simulink model "Rocket_Full_Simulation"  (R2022b)
settings: Solver=VariableStepAuto  StartTime=0.0  StopTime=5  FixedStep=0.001  EnableMultiTasking=on
model workspace (MAT data in the model file):
  Length_NC = Simulink.Parameter
  Length_NC.DataType = 'auto'
  Length_NC.Complexity = 'real'
  Length_NC.Dimensions = [0 0]
undefined symbols (not defined in the file): sigbuilder_block
libraries: simulink_extras x3, simulink x3, sharedtransform x2, mspsensorlib x1, aerolibatmos2 x1, vrlib x1
settings Model: Creator=Poseidon  LastModifiedBy=Poseidon
settings SolverCC: MaxConsecutiveMinStep=3  ZeroCrossAlgorithm=Adaptive  AutoInsertRateTranBlk=on
settings DataIOCC: Refine=2
settings DebuggingCC: ReadBeforeWriteMsg=DisableAll  WriteAfterWriteMsg=DisableAll  WriteAfterReadMsg=DisableAll  MaskedZcDiagnostic=none  IgnoredZcDiagnostic=none  MultiTaskDSMMsg=none
settings ModelReferenceCC: UpdateModelReferenceTargets=IfOutOfDate  EnableRefExpFcnMdlSchedulingChecks=on
settings SFSimCC: SFSimEcho=off

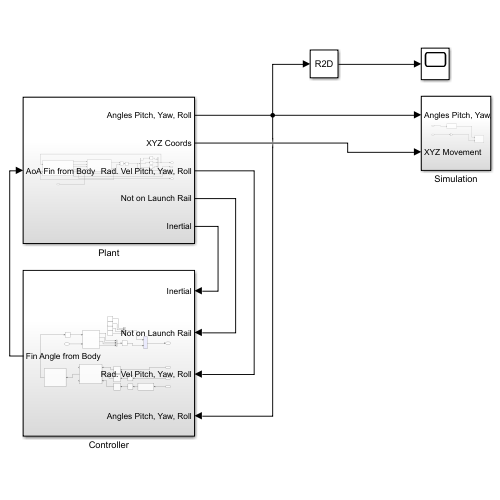
[thumbnail: Simulink's stored preview of the top-level diagram]
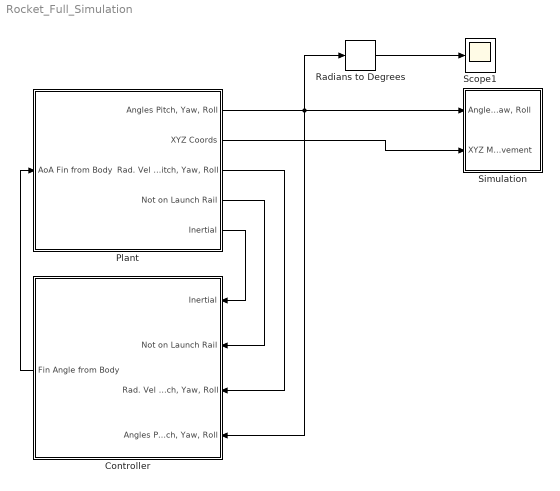
== system Rocket_Full_Simulation ==
  Controller : Subsystem
  Plant : Subsystem
  Radians to Degrees : simulink_extras/Transformations/Radians to Degrees
  Scope1 : Scope
  Simulation : Subsystem
  wires:
  Plant/2(XYZ Coords) -> Simulation/2(XYZ Movement)
  Plant/4(Not on Launch Rail) -> Controller/2(Not on Launch Rail)
  Plant/5(Inertial) -> Controller/1(Inertial)
  Controller/1(Fin Angle from Body) -> Plant/1(AoA Fin from Body)
  Plant/1("Angles Pitch, Yaw, Roll") -> Controller/4("Angles Pitch, Yaw, Roll"), Simulation/1("Angles Pitch, Yaw, Roll"), Radians to Degrees/1
  Plant/3("Rad. Vel Pitch, Yaw, Roll") -> Controller/3("Rad. Vel Pitch, Yaw, Roll")
  Radians to Degrees/1 -> Scope1/1

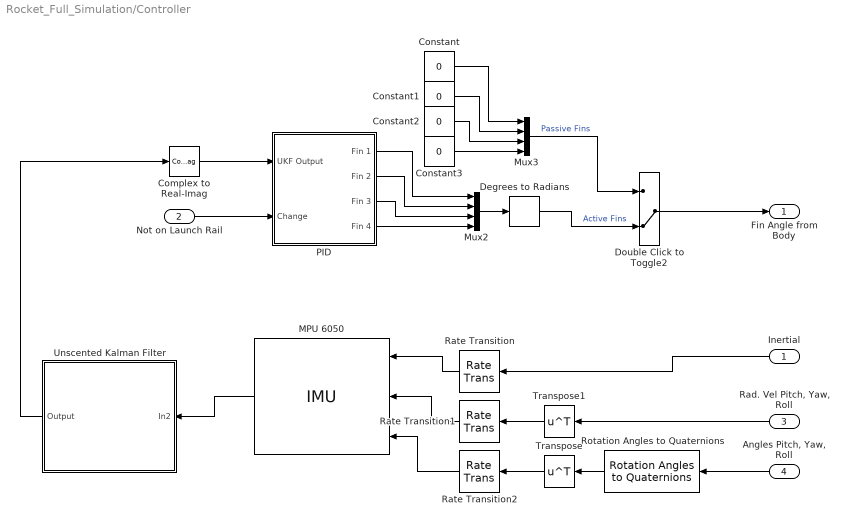
== system Rocket_Full_Simulation/Controller ==
  Inertial : Inport
  Not on Launch Rail : Inport  Port=2
  "Rad. Vel Pitch, Yaw, Roll" : Inport  Port=3
  "Angles Pitch, Yaw, Roll" : Inport  Port=4
  Complex to Real-Imag : ComplexToRealImag  Output=Real
  Constant{,1..3} (4 alike) : Constant  Value=0
  Degrees to Radians : simulink_extras/Transformations/Degrees to Radians
  Double Click to Toggle2 : ManualSwitch  CurrentSetting=0
  MPU 6050 : mspsensorlib/IMU  DispRefFrame=NED  Temperature=25  MagneticFieldNED=[ 27.5550, -2.4169, -16.0849 ]  MagneticFieldENU=[ -2.4169, 27.5550, 16.0849 ]  SeedDouble=67  SimulateUsing=Code generation  AccelParamsMeasurementRange=160  AccelParamsResolution=0.00479  AccelParamsConstantBias=[ 0, 0, 0 ]  AccelParamsAxesMisalignment=[ 100, 0, 0; 0, 100, 0; 0, 0, 100 ]  AccelParamsNoiseDensity=[ 0, 0, 0 ]  AccelParamsBiasInstability=[ 0, 0, 0 ]  AccelParamsRandomWalk=[ 0, 0, 0 ]  AccelParamsTemperatureBias=[ 0, 0, 0 ]  AccelParamsTemperatureScaleFactor=[ 0, 0, 0 ]  GyroParamsMeasurementRange=4.36332  GyroParamsResolution=0.000133157958984  GyroParamsConstantBias=[ 0, 0, 0 ]  GyroParamsAxesMisalignment=[ 100, 0, 0; 0, 100, 0; 0, 0, 100 ]  GyroParamsAccelerationBias=[ 0, 0, 0 ]  GyroParamsNoiseDensity=[ 5.24*10^-5, 5.24*10^-5, 5.24*10^-5 ]  GyroParamsBiasInstability=[ 2.09*10^-5, 2.09*10^-5, 2.09*10^-5 ]  GyroParamsRandomWalk=[ 0, 0, 0 ]  GyroParamsTemperatureBias=[ 0, 0, 0 ]  GyroParamsTemperatureScaleFactor=[ 0, 0, 0 ]  MagParamsMeasurementRange=Inf  MagParamsResolution=0  MagParamsConstantBias=[ 0, 0, 0 ]  MagParamsAxesMisalignment=[ 100, 0, 0; 0, 100, 0; 0, 0, 100 ]  MagParamsNoiseDensity=[ 0, 0, 0 ]  MagParamsBiasInstability=[ 0, 0, 0 ]  MagParamsRandomWalk=[ 0, 0, 0 ]  MagParamsTemperatureBias=[ 0, 0, 0 ]  MagParamsTemperatureScaleFactor=[ 0, 0, 0 ]
  Mux2 : Mux
  Mux3 : Mux
  PID : Subsystem
  Rate Transition : RateTransition  OutPortSampleTime=0.001
  Rate Transition1 : RateTransition  OutPortSampleTime=0.001
  Rate Transition2 : RateTransition  OutPortSampleTime=0.001
  Rotation Angles to Quaternions : sharedtransform/Rotation Angles to Quaternions  rotationOrder=YZX  aMode=aMode
  Transpose : Math  Operator=transpose
  Transpose1 : Math  Operator=transpose
  Unscented Kalman Filter : Subsystem
  Fin Angle from Body : Outport
  wires:
  Constant3/1 -> Mux3/4
  PID/1(Fin 1) -> Mux2/1
  Mux2/1 -> Degrees to Radians/1
  PID/4(Fin 4) -> Mux2/4
  Constant2/1 -> Mux3/3
  Constant/1 -> Mux3/1
  PID/3(Fin 3) -> Mux2/3
  PID/2(Fin 2) -> Mux2/2
  Mux3/1 -> Double Click to Toggle2/1  "Passive Fins"
  Constant1/1 -> Mux3/2
  Complex to Real-Imag/1 -> PID/1(UKF Output)
  Unscented Kalman Filter/1(Output) -> Complex to Real-Imag/1
  Degrees to Radians/1 -> Double Click to Toggle2/2  "Active Fins"
  Double Click to Toggle2/1 -> Fin Angle from Body/1
  Not on Launch Rail/1 -> PID/2(Change)
  "Rad. Vel Pitch, Yaw, Roll"/1 -> Transpose1/1
  "Angles Pitch, Yaw, Roll"/1 -> Rotation Angles to Quaternions/1
  MPU 6050/2 -> Unscented Kalman Filter/1(In2)
  Inertial/1 -> Rate Transition/1
  Transpose/1 -> Rate Transition2/1
  Rate Transition2/1 -> MPU 6050/3
  Rate Transition/1 -> MPU 6050/1
  Rotation Angles to Quaternions/1 -> Transpose/1
  Rate Transition1/1 -> MPU 6050/2
  Transpose1/1 -> Rate Transition1/1

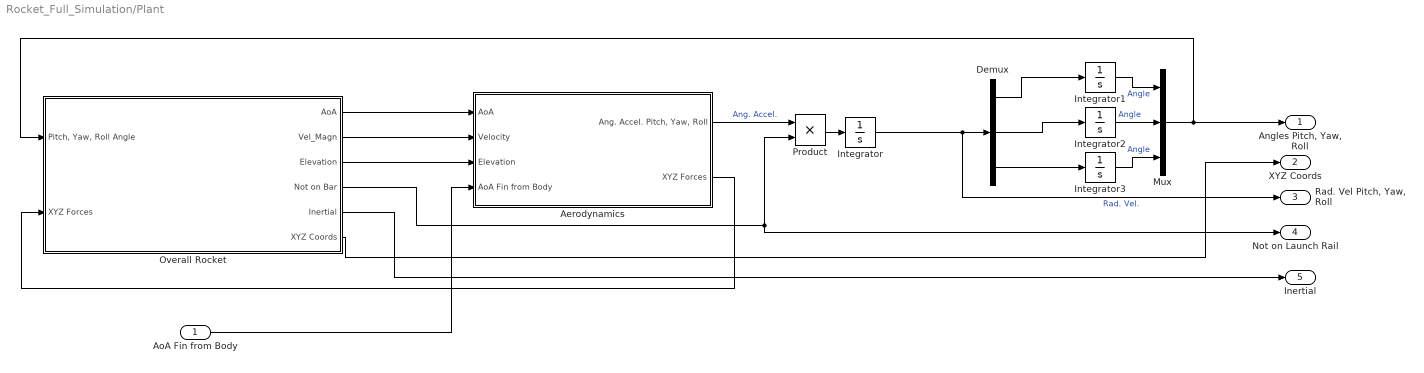
== system Rocket_Full_Simulation/Plant ==
  AoA Fin from Body : Inport
  Aerodynamics : Subsystem
  Demux : Demux  Outputs=3
  Integrator : Integrator
  Integrator1 : Integrator  InitialCondition=0*(pi/180)
  Integrator2 : Integrator
  Integrator3 : Integrator
  Mux : Mux  Inputs=3
  Overall Rocket : Subsystem
  Product : Product
  "Angles Pitch, Yaw, Roll" : Outport
  XYZ Coords : Outport  Port=2
  "Rad. Vel Pitch, Yaw, Roll" : Outport  Port=3
  Not on Launch Rail : Outport  Port=4
  Inertial : Outport  Port=5
  wires:
  Integrator2/1 -> Mux/2  "Angle"
  Product/1 -> Integrator/1
  Integrator/1 -> "Rad. Vel Pitch, Yaw, Roll"/1, Demux/1  "Rad. Vel."
  Demux/2 -> Integrator2/1
  Demux/1 -> Integrator1/1
  Integrator3/1 -> Mux/3  "Angle"
  Demux/3 -> Integrator3/1
  Integrator1/1 -> Mux/1  "Angle"
  Mux/1 -> Overall Rocket/1("Pitch, Yaw, Roll Angle"), "Angles Pitch, Yaw, Roll"/1
  AoA Fin from Body/1 -> Aerodynamics/4(AoA Fin from Body)
  Overall Rocket/1(AoA) -> Aerodynamics/1(AoA)
  Overall Rocket/5(Inertial) -> Inertial/1
  Overall Rocket/2(Vel_Magn) -> Aerodynamics/2(Velocity)
  Overall Rocket/3(Elevation) -> Aerodynamics/3(Elevation)
  Overall Rocket/4(Not on Bar) -> Not on Launch Rail/1, Product/2
  Aerodynamics/1("Ang. Accel. Pitch, Yaw, Roll") -> Product/1  "Ang. Accel."
  Aerodynamics/2(XYZ Forces) -> Overall Rocket/2(XYZ Forces)
  Overall Rocket/6(XYZ Coords) -> XYZ Coords/1

== system Rocket_Full_Simulation/Simulation ==
  note: Convert to coordinates for simulation
  "Angles Pitch, Yaw, Roll" : Inport
  XYZ Movement : Inport  Port=2
  MATLAB Function : MATLAB Function  TreatAsAtomicUnit=on
  Multiply : Gain  Gain=0
  VR Sink : vrlib/VR Sink  InstantiateOnLoad=on  SampleTime=0.1  ViewEnable=on  RemoteChange=off  RemoteView=off  FieldsWritten=node_Transform.rotation.4.1.1.double#node_Transform.translation.3.1.1.double  WorldFileName=C:\Users\Trenton VerKuilen\OneDrive - lmu.edu\School\Capstone\2Stage_Rocket.wrl  AutoView=off  VideoDimensions=[]  AllowVariableSize=off
  wires:
  XYZ Movement/1 -> Multiply/1
  Multiply/1 -> VR Sink/2
  "Angles Pitch, Yaw, Roll"/1 -> MATLAB Function/1(Angles)
  MATLAB Function/1(Rotation) -> VR Sink/1

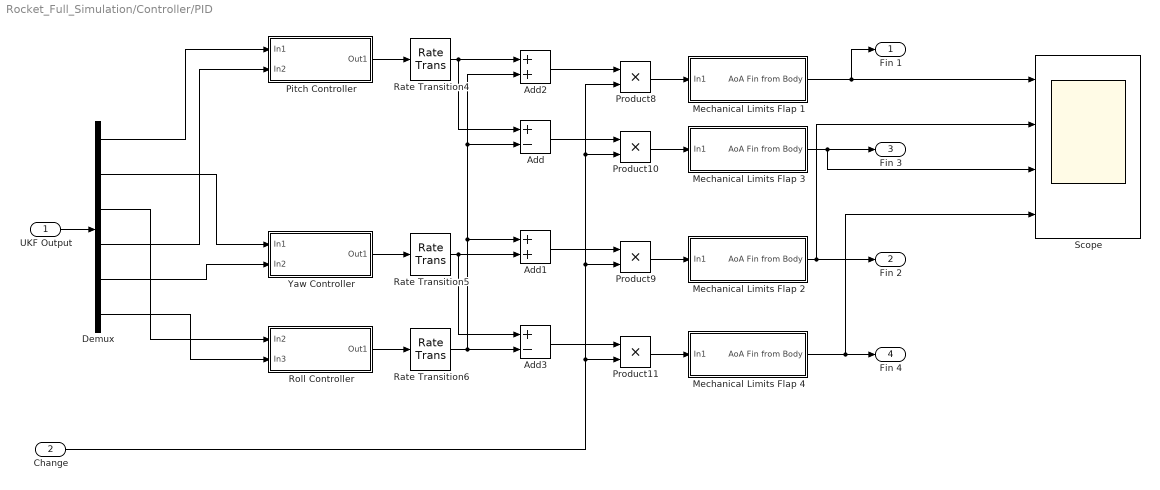
== system Rocket_Full_Simulation/Controller/PID ==
  UKF Output : Inport
  Change : Inport  Port=2
  Add : Sum  Inputs=+-
  Add1 : Sum
  Add2 : Sum
  Add3 : Sum  Inputs=+-
  Demux : Demux  Outputs=6
  Mechanical Limits Flap 1 : Subsystem
  Mechanical Limits Flap 2 : Subsystem
  Mechanical Limits Flap 3 : Subsystem
  Mechanical Limits Flap 4 : Subsystem
  Pitch Controller : Subsystem
  Product{8..11} (4 alike) : Product
  Rate Transition4 : RateTransition
  Rate Transition5 : RateTransition
  Rate Transition6 : RateTransition
  Roll Controller : Subsystem
  Scope : Scope  NumInputPorts=4
  Yaw Controller : Subsystem
  Fin 1 : Outport
  Fin 2 : Outport  Port=2
  Fin 3 : Outport  Port=3
  Fin 4 : Outport  Port=4
  wires:
  UKF Output/1 -> Demux/1
  Demux/5 -> Yaw Controller/2(In2)
  Demux/2 -> Yaw Controller/1(In1)
  Demux/1 -> Pitch Controller/1(In1)
  Pitch Controller/1(Out1) -> Rate Transition4/1
  Demux/3 -> Roll Controller/1(In2)
  Demux/4 -> Pitch Controller/2(In2)
  Demux/6 -> Roll Controller/2(In3)
  Yaw Controller/1(Out1) -> Rate Transition5/1
  Roll Controller/1(Out1) -> Rate Transition6/1
  Rate Transition4/1 -> Add/1, Add2/1
  Rate Transition5/1 -> Add3/1, Add1/2
  Rate Transition6/1 -> Add2/2, Add/2, Add1/1, Add3/2
  Add2/1 -> Product8/1
  Add/1 -> Product10/1
  Add1/1 -> Product9/1
  Mechanical Limits Flap 2/1(AoA Fin from Body) -> Scope/2, Fin 2/1
  Change/1 -> Product8/2, Product10/2, Product9/2, Product11/2
  Add3/1 -> Product11/1
  Product8/1 -> Mechanical Limits Flap 1/1(In1)
  Product9/1 -> Mechanical Limits Flap 2/1(In1)
  Product10/1 -> Mechanical Limits Flap 3/1(In1)
  Product11/1 -> Mechanical Limits Flap 4/1(In1)
  Mechanical Limits Flap 1/1(AoA Fin from Body) -> Fin 1/1, Scope/1
  Mechanical Limits Flap 3/1(AoA Fin from Body) -> Scope/3, Fin 3/1
  Mechanical Limits Flap 4/1(AoA Fin from Body) -> Scope/4, Fin 4/1

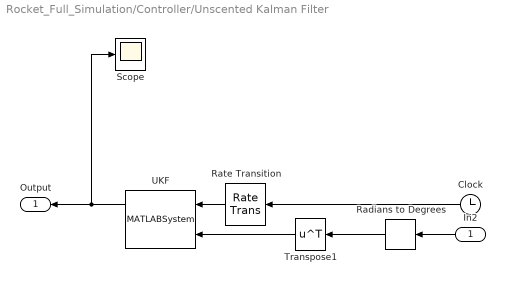
== system Rocket_Full_Simulation/Controller/Unscented Kalman Filter ==
  In2 : Inport
  Clock : Clock
  Radians to Degrees : simulink_extras/Transformations/Radians to Degrees
  Rate Transition : RateTransition  OutPortSampleTime=0.001
  Scope : Scope
  Transpose1 : Math  Operator=transpose
  UKF : MATLABSystem  System=UKF  kappa=0.0  alfa=0.001  beta=2.0  x_0=0  Q_=0.1  R_=0.1  SimulateUsing=Code generation
      mask Type: UKF
      mask Display:
      | disp('UKF');
      | port_label('input',1,'time');
      | port_label('input',2,'z');
      | port_label('output',1,'y');
      | port_label('output',2,'P');
  Output : Outport
  wires:
  UKF/1 -> Scope/1, Output/1
  In2/1 -> Radians to Degrees/1
  Radians to Degrees/1 -> Transpose1/1
  Transpose1/1 -> UKF/2
  Clock/1 -> Rate Transition/1
  Rate Transition/1 -> UKF/1

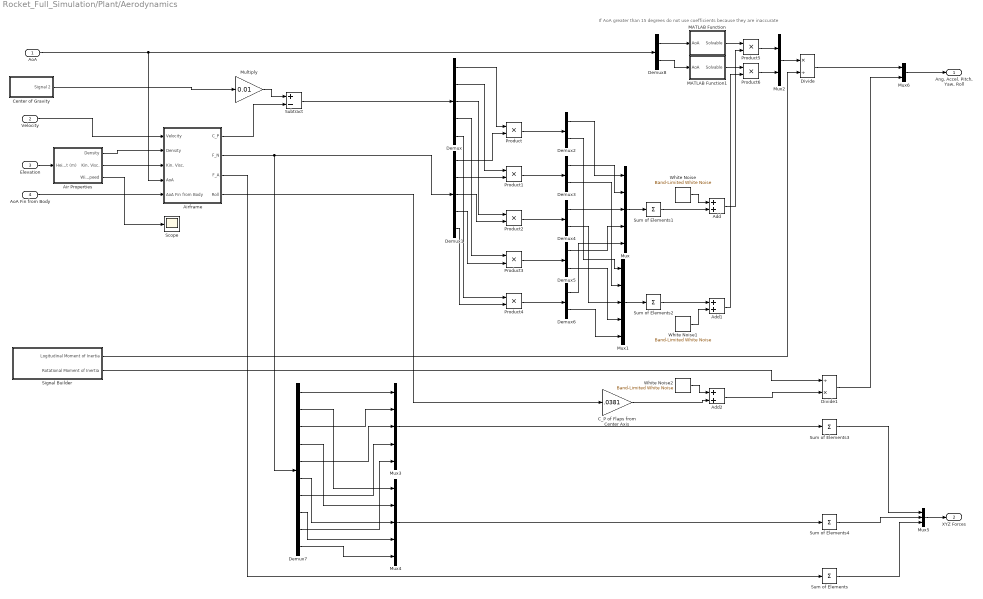
== system Rocket_Full_Simulation/Plant/Aerodynamics ==
  note: If AoA greater than 15 degrees do not use coefficients because they are inaccurate
  AoA : Inport
  Velocity : Inport  Port=2
  Elevation : Inport  Port=3
  AoA Fin from Body : Inport  Port=4
  Add : Sum
  Add1 : Sum
  Add2 : Sum
  Air Properties : Subsystem
  Airframe : Subsystem
  C_P of Flaps from Center Axis : Gain  Gain=.0381
  Center of Gravity : Subsystem  Tag=STV Subsys  LoadFcn=sigbuilder_block('load');  StartFcn=sigbuilder_block('start');  StopFcn=sigbuilder_block('stop');  ClipboardFcn=sigbuilder_block('clipboard');  mask(Sigbuilder block){tuvar=[0:10]}
      mask help: Simulink:masks:SigbuilderBlock_MD
      mask init:
      | if ~strcmp(get_param(bdroot(gcbh),'SimulationStatus'),'stopped') tuvar = sigbuilder_block('maskInit'); end
      settings: CopyFcn=sigbuilder_block('copy');  DeleteFcn=sigbuilder_block('delete');  ModelCloseFcn=sigbuilder_block('modelClose');  PreSaveFcn=sigbuilder_block('preSave');  PauseFcn=sigbuilder_block('pause');  ContinueFcn=sigbuilder_block('continue');  NameChangeFcn=sigbuilder_block('namechange');  OpenFcn=sigbuilder_block('open',[309.6 144.6 550.8 400.2 ]);  CloseFcn=sigbuilder_block('close');
      mask Display: plot(0, 0, 100, 100,[2, 2, 32, 32, 2], [68, 8, 8, 68, 68],[32, 2], [38, 38], [32, 19, 2],[53, 60, 44], [32, 17, 17, 2],[16, 16, 31, 31]);txt = getActiveGroup(gcbh);text(2, 100, txt,'verticalAlignment', 'top');
  Demux : Demux  Outputs=5
  Demux1 : Demux  Outputs=5
  Demux{2..6,8} (6 alike) : Demux  Outputs=2
  Demux7 : Demux  Outputs=10
  Divide : Product  Inputs=*/
  Divide1 : Product  Inputs=/*
  MATLAB Function : MATLAB Function  TreatAsAtomicUnit=on
  MATLAB Function1 : MATLAB Function  TreatAsAtomicUnit=on
  Multiply : Gain  Gain=0.01
  Mux{,1,3..4} (4 alike) : Mux  Inputs=5
  Mux2 : Mux  Inputs=2
  Mux5 : Mux  Inputs=3
  Mux6 : Mux  Inputs=2
  Product{,1..6} (7 alike) : Product
  Scope : Scope
  Signal Builder : Subsystem  Tag=STV Subsys  LoadFcn=sigbuilder_block('load');  StartFcn=sigbuilder_block('start');  StopFcn=sigbuilder_block('stop');  ClipboardFcn=sigbuilder_block('clipboard');  mask(Sigbuilder block){tuvar=[0:10]}
      mask help: Simulink:masks:SigbuilderBlock_MD
      mask init:
      | if ~strcmp(get_param(bdroot(gcbh),'SimulationStatus'),'stopped') tuvar = sigbuilder_block('maskInit'); end
      settings: CopyFcn=sigbuilder_block('copy');  DeleteFcn=sigbuilder_block('delete');  ModelCloseFcn=sigbuilder_block('modelClose');  PreSaveFcn=sigbuilder_block('preSave');  PauseFcn=sigbuilder_block('pause');  ContinueFcn=sigbuilder_block('continue');  NameChangeFcn=sigbuilder_block('namechange');  OpenFcn=sigbuilder_block('open',[375 140.4 550.8 400.2 ]);  CloseFcn=sigbuilder_block('close');
      mask Display: plot(0, 0, 100, 100,[2, 2, 32, 32, 2], [68, 8, 8, 68, 68],[32, 2], [38, 38], [32, 19, 2],[53, 60, 44], [32, 17, 17, 2],[16, 16, 31, 31]);txt = getActiveGroup(gcbh);text(2, 100, txt,'verticalAlignment', 'top');
  Subtract : Sum  Inputs=+-
  Sum of Elements{,1..4} (5 alike) : Sum  Inputs=+
  White Noise : simulink/Sources/Band-Limited White Noise  Cov=[0.005]  Ts=0.5  seed=[12345]
  White Noise1 : simulink/Sources/Band-Limited White Noise  Cov=[0.005]  Ts=0.5  seed=[84932]
  White Noise2 : simulink/Sources/Band-Limited White Noise  Cov=[0.000001]  Ts=0.5  seed=[86986]
  "Ang. Accel. Pitch, Yaw, Roll" : Outport
  XYZ Forces : Outport  Port=2
  wires:
  Airframe/1(C_P) -> Subtract/2
  Elevation/1 -> Air Properties/1(Height (m))
  Demux7/5 -> Mux3/3
  Center of Gravity/1(Signal 2) -> Multiply/1
  C_P of Flaps from Center Axis/1 -> Add2/2
  AoA Fin from Body/1 -> Airframe/5(AoA Fin from Body)
  AoA/1 -> Demux8/1, Airframe/4(AoA)
  Air Properties/3(Wind Speed) -> Scope/1
  Demux/3 -> Product2/1
  Demux7/8 -> Mux4/4
  Demux8/1 -> MATLAB Function/1(AoA)
  Velocity/1 -> Airframe/1(Velocity)
  Air Properties/2(Kin. Visc.) -> Airframe/3(Kin. Visc.)
  Demux3/2 -> Mux1/2
  Demux/5 -> Product4/1
  Air Properties/1(Density) -> Airframe/2(Density)
  Multiply/1 -> Subtract/1
  Sum of Elements4/1 -> Mux5/2
  Airframe/2(F_N) -> Demux1/1, Demux7/1
  Airframe/3(F_A) -> Sum of Elements/1
  Airframe/4(Roll) -> C_P of Flaps from Center Axis/1
  Demux7/2 -> Mux4/1
  Subtract/1 -> Demux/1
  Demux7/1 -> Mux3/1
  Demux7/3 -> Mux3/2
  Demux7/4 -> Mux4/2
  Demux7/6 -> Mux4/3
  Demux6/2 -> Mux1/5
  Demux7/7 -> Mux3/4
  Demux7/9 -> Mux3/5
  Product4/1 -> Demux6/1
  Mux3/1 -> Sum of Elements3/1
  Demux7/10 -> Mux4/5
  Demux1/4 -> Product3/2
  Mux1/1 -> Sum of Elements2/1
  Add2/1 -> Divide1/2
  White Noise2/1 -> Add2/1
  Demux/1 -> Product/1
  Demux/2 -> Product1/1
  Sum of Elements3/1 -> Mux5/1
  Demux/4 -> Product3/1
  Demux4/1 -> Mux/3
  Demux1/1 -> Product/2
  Demux1/2 -> Product1/2
  Demux1/3 -> Product2/2
  Product3/1 -> Demux5/1
  Demux1/5 -> Product4/2
  Mux4/1 -> Sum of Elements4/1
  Signal Builder/1(Logitudinal Moment of Inertia) -> Divide/2
  White Noise/1 -> Add/1
  Signal Builder/2(Rotational Moment of Inertia) -> Divide1/1
  Demux3/1 -> Mux/2
  Product/1 -> Demux2/1
  Product1/1 -> Demux3/1
  Demux5/1 -> Mux/4
  Product2/1 -> Demux4/1
  Divide1/1 -> Mux6/2
  Demux2/1 -> Mux/1
  Demux2/2 -> Mux1/1
  Demux4/2 -> Mux1/3
  Demux5/2 -> Mux1/4
  Demux6/1 -> Mux/5
  Mux/1 -> Sum of Elements1/1
  Demux8/2 -> MATLAB Function1/1(AoA)
  Sum of Elements1/1 -> Add/2
  Sum of Elements2/1 -> Add1/1
  White Noise1/1 -> Add1/2
  MATLAB Function/1(Solvable) -> Product5/1
  Add/1 -> Product5/2
  MATLAB Function1/1(Solvable) -> Product6/1
  Add1/1 -> Product6/2
  Product5/1 -> Mux2/1
  Product6/1 -> Mux2/2
  Mux2/1 -> Divide/1
  Mux5/1 -> XYZ Forces/1
  Mux6/1 -> "Ang. Accel. Pitch, Yaw, Roll"/1
  Divide/1 -> Mux6/1
  Sum of Elements/1 -> Mux5/3

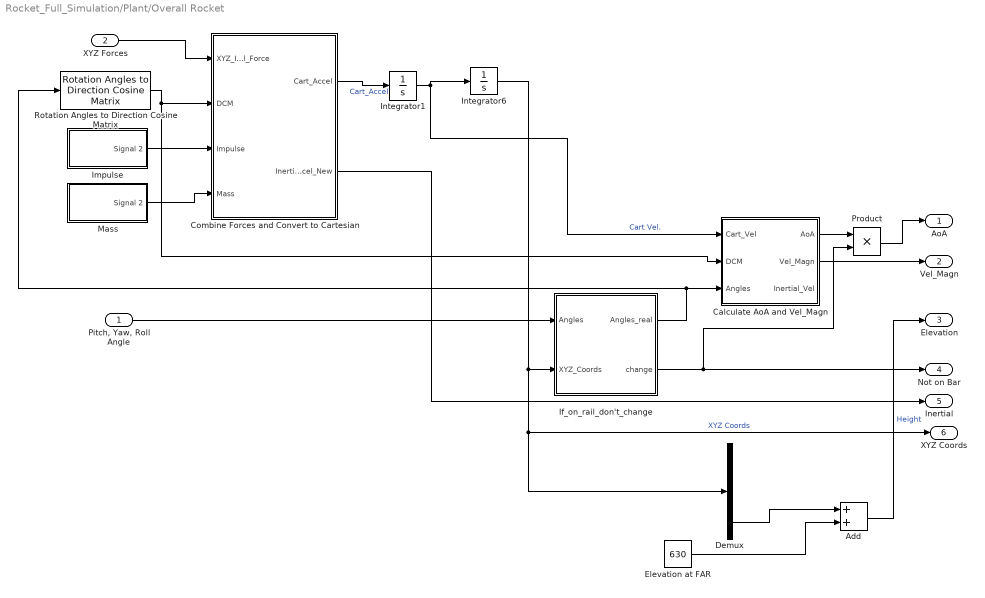
== system Rocket_Full_Simulation/Plant/Overall Rocket ==
  "Pitch, Yaw, Roll Angle" : Inport
  XYZ Forces : Inport  Port=2
  Add : Sum
  Calculate AoA and Vel_Magn : MATLAB Function  TreatAsAtomicUnit=on
  Combine Forces and Convert to Cartesian : MATLAB Function  TreatAsAtomicUnit=on
  Demux : Demux  Outputs=3
  Elevation at FAR : Constant  Value=630
  If_on_rail_don't_change : MATLAB Function  TreatAsAtomicUnit=on
  Impulse : Subsystem  Tag=STV Subsys  LoadFcn=sigbuilder_block('load');  StartFcn=sigbuilder_block('start');  StopFcn=sigbuilder_block('stop');  ClipboardFcn=sigbuilder_block('clipboard');  mask(Sigbuilder block){tuvar=[0:10]}
      mask help: Simulink:masks:SigbuilderBlock_MD
      mask init:
      | if ~strcmp(get_param(bdroot(gcbh),'SimulationStatus'),'stopped') tuvar = sigbuilder_block('maskInit'); end
      settings: CopyFcn=sigbuilder_block('copy');  DeleteFcn=sigbuilder_block('delete');  ModelCloseFcn=sigbuilder_block('modelClose');  PreSaveFcn=sigbuilder_block('preSave');  PauseFcn=sigbuilder_block('pause');  ContinueFcn=sigbuilder_block('continue');  NameChangeFcn=sigbuilder_block('namechange');  OpenFcn=sigbuilder_block('open',[396 -4.2 574.2 590.4 ]);  CloseFcn=sigbuilder_block('close');
      mask Display: plot(0, 0, 100, 100,[2, 2, 32, 32, 2], [68, 8, 8, 68, 68],[32, 2], [38, 38], [32, 19, 2],[53, 60, 44], [32, 17, 17, 2],[16, 16, 31, 31]);txt = getActiveGroup(gcbh);text(2, 100, txt,'verticalAlignment', 'top');
  Integrator1 : Integrator  IgnoreLimit=on
  Integrator6 : Integrator
  Mass : Subsystem  Tag=STV Subsys  LoadFcn=sigbuilder_block('load');  StartFcn=sigbuilder_block('start');  StopFcn=sigbuilder_block('stop');  ClipboardFcn=sigbuilder_block('clipboard');  mask(Sigbuilder block){tuvar=[0:10]}
      mask help: Simulink:masks:SigbuilderBlock_MD
      mask init:
      | if ~strcmp(get_param(bdroot(gcbh),'SimulationStatus'),'stopped') tuvar = sigbuilder_block('maskInit'); end
      settings: CopyFcn=sigbuilder_block('copy');  DeleteFcn=sigbuilder_block('delete');  ModelCloseFcn=sigbuilder_block('modelClose');  PreSaveFcn=sigbuilder_block('preSave');  PauseFcn=sigbuilder_block('pause');  ContinueFcn=sigbuilder_block('continue');  NameChangeFcn=sigbuilder_block('namechange');  OpenFcn=sigbuilder_block('open',[424.8 154.2 550.8 400.2 ]);  CloseFcn=sigbuilder_block('close');
      mask Display: plot(0, 0, 100, 100,[2, 2, 32, 32, 2], [68, 8, 8, 68, 68],[32, 2], [38, 38], [32, 19, 2],[53, 60, 44], [32, 17, 17, 2],[16, 16, 31, 31]);txt = getActiveGroup(gcbh);text(2, 100, txt,'verticalAlignment', 'top');
  Product : Product
  Rotation Angles to Direction Cosine Matrix : sharedtransform/Rotation Angles to Direction Cosine Matrix  rotationOrder=YZX  aMode=aMode
  AoA : Outport
  Vel_Magn : Outport  Port=2
  Elevation : Outport  Port=3
  Not on Bar : Outport  Port=4
  Inertial : Outport  Port=5
  XYZ Coords : Outport  Port=6
  wires:
  XYZ Forces/1 -> Combine Forces and Convert to Cartesian/1(XYZ_Inertial_Force)
  Impulse/1(Signal 2) -> Combine Forces and Convert to Cartesian/3(Impulse)
  Rotation Angles to Direction Cosine Matrix/1 -> Calculate AoA and Vel_Magn/2(DCM), Combine Forces and Convert to Cartesian/2(DCM)
  Integrator1/1 -> Integrator6/1, Calculate AoA and Vel_Magn/1(Cart_Vel)  "Cart Vel."
  Mass/1(Signal 2) -> Combine Forces and Convert to Cartesian/4(Mass)
  Combine Forces and Convert to Cartesian/2(Inertial_Accel_New) -> Inertial/1
  Combine Forces and Convert to Cartesian/1(Cart_Accel) -> Integrator1/1  "Cart_Accel"
  Integrator6/1 -> Demux/1, XYZ Coords/1, If_on_rail_don't_change/2(XYZ_Coords)  "XYZ Coords"
  "Pitch, Yaw, Roll Angle"/1 -> If_on_rail_don't_change/1(Angles)
  Demux/3 -> Add/1
  Elevation at FAR/1 -> Add/2
  If_on_rail_don't_change/1(Angles_real) -> Rotation Angles to Direction Cosine Matrix/1, Calculate AoA and Vel_Magn/3(Angles)
  If_on_rail_don't_change/2(change) -> Product/2, Not on Bar/1
  Add/1 -> Elevation/1  "Height"
  Calculate AoA and Vel_Magn/2(Vel_Magn) -> Vel_Magn/1
  Calculate AoA and Vel_Magn/1(AoA) -> Product/1
  Product/1 -> AoA/1

== system Rocket_Full_Simulation/Controller/PID/Mechanical Limits Flap 1 ==
  In1 : Inport
  Integrator Limited : Integrator  LimitOutput=on  UpperSaturationLimit=15  LowerSaturationLimit=-15
  Rate Limit : Saturate  UpperLimit=857.14  LowerLimit=-857.14
  Servo Gain : Gain  Gain=6
  Sum2 : Sum  Inputs=|+-
  AoA Fin from Body : Outport
  wires:
  Sum2/1 -> Servo Gain/1
  Servo Gain/1 -> Rate Limit/1
  Rate Limit/1 -> Integrator Limited/1
  In1/1 -> Sum2/1
  Integrator Limited/1 -> AoA Fin from Body/1, Sum2/2

== system Rocket_Full_Simulation/Controller/PID/Mechanical Limits Flap 2 ==
  In1 : Inport
  Integrator Limited : Integrator  LimitOutput=on  UpperSaturationLimit=15  LowerSaturationLimit=-15
  Rate Limit : Saturate  UpperLimit=857.14  LowerLimit=-857.14
  Servo Gain : Gain  Gain=6
  Sum2 : Sum  Inputs=|+-
  AoA Fin from Body : Outport
  wires:
  Sum2/1 -> Servo Gain/1
  Servo Gain/1 -> Rate Limit/1
  Rate Limit/1 -> Integrator Limited/1
  In1/1 -> Sum2/1
  Integrator Limited/1 -> AoA Fin from Body/1, Sum2/2

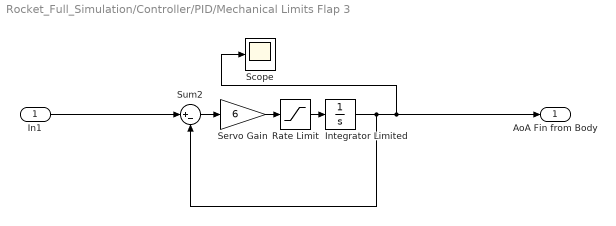
== system Rocket_Full_Simulation/Controller/PID/Mechanical Limits Flap 3 ==
  In1 : Inport
  Integrator Limited : Integrator  LimitOutput=on  UpperSaturationLimit=15  LowerSaturationLimit=-15
  Rate Limit : Saturate  UpperLimit=857.14  LowerLimit=-857.14
  Scope : Scope
  Servo Gain : Gain  Gain=6
  Sum2 : Sum  Inputs=|+-
  AoA Fin from Body : Outport
  wires:
  Sum2/1 -> Servo Gain/1
  Servo Gain/1 -> Rate Limit/1
  Rate Limit/1 -> Integrator Limited/1
  In1/1 -> Sum2/1
  Integrator Limited/1 -> Scope/1, AoA Fin from Body/1, Sum2/2

== system Rocket_Full_Simulation/Controller/PID/Mechanical Limits Flap 4 ==
  In1 : Inport
  Integrator Limited : Integrator  LimitOutput=on  UpperSaturationLimit=15  LowerSaturationLimit=-15
  Rate Limit : Saturate  UpperLimit=857.14  LowerLimit=-857.14
  Servo Gain : Gain  Gain=6
  Sum2 : Sum  Inputs=|+-
  AoA Fin from Body : Outport
  wires:
  Sum2/1 -> Servo Gain/1
  Servo Gain/1 -> Rate Limit/1
  Rate Limit/1 -> Integrator Limited/1
  In1/1 -> Sum2/1
  Integrator Limited/1 -> AoA Fin from Body/1, Sum2/2

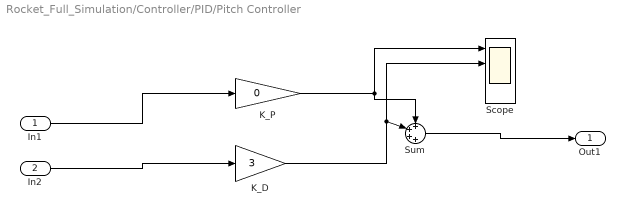
== system Rocket_Full_Simulation/Controller/PID/Pitch Controller ==
  In1 : Inport
  In2 : Inport  Port=2
  K_D : Gain  Gain=3
  K_P : Gain  Gain=0
  Scope : Scope  NumInputPorts=4
  Sum : Sum  Inputs=++++
  Out1 : Outport
  wires:
  In2/1 -> K_D/1
  In1/1 -> K_P/1
  K_P/1 -> Sum/1, Scope/1
  K_D/1 -> Scope/2, Sum/2
  Sum/1 -> Out1/1

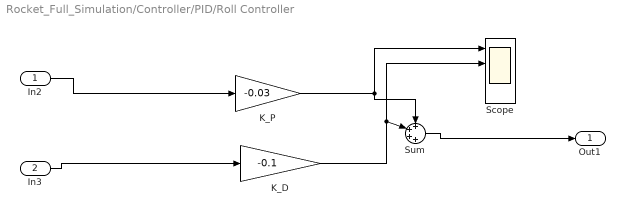
== system Rocket_Full_Simulation/Controller/PID/Roll Controller ==
  In2 : Inport
  In3 : Inport  Port=2
  K_D : Gain  Gain=-0.1
  K_P : Gain  Gain=-0.03
  Scope : Scope  NumInputPorts=4
  Sum : Sum  Inputs=++++
  Out1 : Outport
  wires:
  In3/1 -> K_D/1
  K_P/1 -> Sum/1, Scope/1
  K_D/1 -> Scope/2, Sum/2
  In2/1 -> K_P/1
  Sum/1 -> Out1/1

== system Rocket_Full_Simulation/Controller/PID/Yaw Controller ==
  In1 : Inport
  In2 : Inport  Port=2
  K_D : Gain  Gain=3
  K_P : Gain  Gain=0
  Scope : Scope  NumInputPorts=4
  Sum : Sum  Inputs=++++
  Out1 : Outport
  wires:
  In1/1 -> K_P/1
  K_P/1 -> Sum/1, Scope/1
  K_D/1 -> Scope/2, Sum/2
  Sum/1 -> Out1/1
  In2/1 -> K_D/1

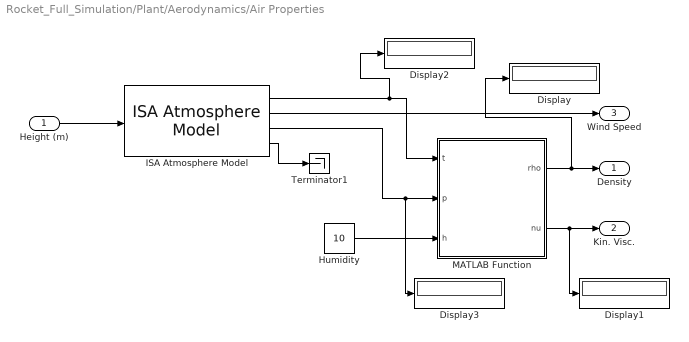
== system Rocket_Full_Simulation/Plant/Aerodynamics/Air Properties ==
  Height (m) : Inport
  Display{,1..3} (4 alike) : Display
  Humidity : Constant  Value=10
  ISA Atmosphere Model : aerolibatmos2/ISA Atmosphere Model  custom=off  g=9.80665  gamma=1.4  R=287.0531  L=0.0065  h_trop=11000  h_strat=20000  rho0=1.225  P0=101325  T0=288.15  h0=0
  MATLAB Function : MATLAB Function  TreatAsAtomicUnit=on
  Terminator1 : Terminator
  Density : Outport
  Kin. Visc. : Outport  Port=2
  Wind Speed : Outport  Port=3
  wires:
  MATLAB Function/2(nu) -> Display1/1, Kin. Visc./1
  MATLAB Function/1(rho) -> Display/1, Density/1
  Humidity/1 -> MATLAB Function/3(h)
  ISA Atmosphere Model/1 -> Display2/1, MATLAB Function/1(t)
  ISA Atmosphere Model/3 -> Display3/1, MATLAB Function/2(p)
  Height (m)/1 -> ISA Atmosphere Model/1
  ISA Atmosphere Model/2 -> Wind Speed/1
  ISA Atmosphere Model/4 -> Terminator1/1

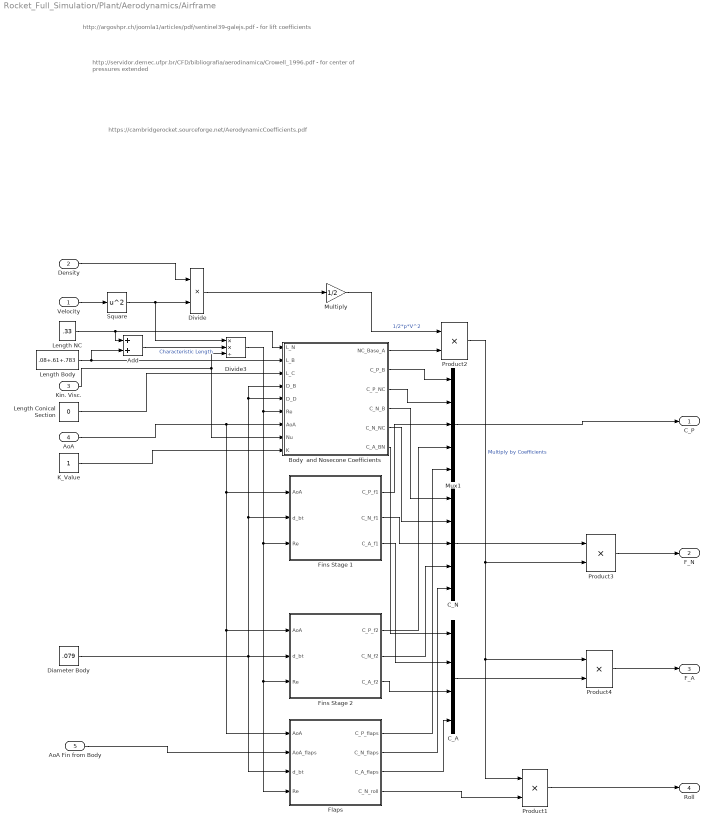
== system Rocket_Full_Simulation/Plant/Aerodynamics/Airframe ==
  note: https://cambridgerocket.sourceforge.net/AerodynamicCoefficients.pdf
  note: http://servidor.demec.ufpr.br/CFD/bibliografia/aerodinamica/Crowell_1996.pdf - for center of pressures extended
  note: http://argoshpr.ch/joomla1/articles/pdf/sentinel39-galejs.pdf - for lift coefficients
  Velocity : Inport
  Density : Inport  Port=2
  Kin. Visc. : Inport  Port=3
  AoA : Inport  Port=4
  AoA Fin from Body : Inport  Port=5
  Add : Sum
  Body  and Nosecone Coefficients : MATLAB Function  TreatAsAtomicUnit=on
  C_A : Mux
  C_N : Mux  Inputs=5
  Diameter Body : Constant  Value=.079
  Divide : Product  Inputs=**
  Divide3 : Product  Inputs=**/
  Fins Stage 1 : MATLAB Function  TreatAsAtomicUnit=on
  Fins Stage 2 : MATLAB Function  TreatAsAtomicUnit=on
  Flaps : MATLAB Function  TreatAsAtomicUnit=on
  K_Value : Constant
  Length Body : Constant  Value=.08+.61+.783
  Length Conical Section : Constant  Value=0
  Length NC : Constant  Value=.33
  Multiply : Gain  Gain=1/2
  Mux1 : Mux  Inputs=5
  Product{1..4} (4 alike) : Product
  Square : Math  Operator=square
  C_P : Outport
  F_N : Outport  Port=2
  F_A : Outport  Port=3
  Roll : Outport  Port=4
  wires:
  Velocity/1 -> Square/1
  Add/1 -> Divide3/2  "Characteristic Length"
  Product2/1 -> Product1/1, Product4/1, Product3/2  "Multiply by Coefficients"
  Length NC/1 -> Add/1, Body  and Nosecone Coefficients/1(L_N)
  Kin. Visc./1 -> Body  and Nosecone Coefficients/8(Nu), Divide3/3
  Length Body/1 -> Add/2, Body  and Nosecone Coefficients/2(L_B)
  Divide/1 -> Multiply/1
  Density/1 -> Divide/1
  AoA/1 -> Flaps/1(AoA), Fins Stage 2/1(AoA), Fins Stage 1/1(AoA), Body  and Nosecone Coefficients/7(AoA)
  Square/1 -> Divide3/1, Divide/2
  C_N/1 -> Product3/1
  Body  and Nosecone Coefficients/4(C_N_B) -> C_N/1
  Length Conical Section/1 -> Body  and Nosecone Coefficients/3(L_C)
  K_Value/1 -> Body  and Nosecone Coefficients/9(K)
  Diameter Body/1 -> Body  and Nosecone Coefficients/5(D_D), Body  and Nosecone Coefficients/4(D_B), Fins Stage 1/2(d_bt), Flaps/3(d_bt), Fins Stage 2/2(d_bt)
  Fins Stage 2/1(C_P_f2) -> Mux1/4
  Divide3/1 -> Flaps/4(Re), Fins Stage 2/3(Re), Fins Stage 1/3(Re), Body  and Nosecone Coefficients/6(Re)
  Flaps/3(C_A_flaps) -> C_A/4
  Multiply/1 -> Product2/1  "1/2*p*V^2"
  Flaps/1(C_P_flaps) -> Mux1/5
  Body  and Nosecone Coefficients/1(NC_Base_A) -> Product2/2
  Body  and Nosecone Coefficients/6(C_A_BN) -> C_A/1
  Body  and Nosecone Coefficients/5(C_N_NC) -> C_N/2
  C_A/1 -> Product4/2
  Fins Stage 2/2(C_N_f2) -> C_N/4
  Fins Stage 2/3(C_A_f2) -> C_A/3
  Flaps/2(C_N_flaps) -> C_N/5
  Mux1/1 -> C_P/1
  Product3/1 -> F_N/1
  Product4/1 -> F_A/1
  Fins Stage 1/2(C_N_f1) -> C_N/3
  Fins Stage 1/3(C_A_f1) -> C_A/2
  Body  and Nosecone Coefficients/3(C_P_NC) -> Mux1/2
  Body  and Nosecone Coefficients/2(C_P_B) -> Mux1/1
  Fins Stage 1/1(C_P_f1) -> Mux1/3
  AoA Fin from Body/1 -> Flaps/2(AoA_flaps)
  Flaps/4(C_N_roll) -> Product1/2
  Product1/1 -> Roll/1

== system Rocket_Full_Simulation/Plant/Aerodynamics/Center of Gravity ==
  Demux : Demux  Tag=STV Demux  Outputs=1
      settings: DisplayOption=none
  FromWs : FromWorkspace  Tag=STV FromWs  VariableName=tuvar
      SigBuilderData=|
      | common.afterFinalStr = 'Extrapolate'
      | common.sampleTime = 0
      | dataSet.timeRange = [0 10]
      | dataSet.name = 'Group 1'
      | sbobj.Groups.Name = 'Group 1'
      | sbobj.Groups.Signals.Name = 'Signal 2'
      | sbobj.Groups.Signals.XData = [0 0.01 0.02 0.03 0.04 0.05 0.06 0.07 0.08 0.09 0.1 0.11 0.12 0.13 0.14 0.15 0.16 0.17 0.18 0.19 0.2 0.21 0.22 0.23 0.24 0.25 0.26 0.27 0.28 0.29 0.3 0.31 0.32 0.33 0.34 0.35 0.36 0.37 0.38 0.39 0.4 0.41 0.42 0.43 0.44 0.455 0.4775 0.51125 0.56125 0.61125 0.66125 0.71125 0.76125 0.81125 0.86125 0.91125 0.95226 0.98929 1.029 1.0781 1.1281 1.1781 1.2281 1.2662 1.3014 1.342 1.392 1.442 1.492 1.5386 1.5886 1.6386 1.6886 1.7386 1.7886 1.8386 1.8886 1.9386 1.9886 2.0386 2.0886 2.1386 2.1886 2.2386 2.2886 2.3386 2.3886 2.4386 2.4886 2.5386 2.5886 2.6386 2.6886 2.7386 2.7886 2.8386 2.8886 10]
      | sbobj.Groups.Signals.YData = [103.89 103.89 103.86 103.83 103.81 103.78 103.76 103.73 103.71 103.69 103.66 103.64 103.61 103.59 103.56 103.54 103.51 103.49 103.47 103.44 103.42 103.39 103.37 103.34 103.32 103.29 103.27 103.24 103.22 103.19 103.17 103.14 103.12 103.09 103.07 103.04 103.02 103 102.97 102.94 102.92 102.89 102.87 102.84 102.82 102.79 102.74 102.67 102.56 102.43 102.3 102.18 102.05 101.93 101.8 101.68 101.57 101.47 101.38 101.27 101.15 101.03 100.92 100.82 100.75 100.68 100.6 100.53 100.48 100.44 100.41 100.38 100.37 100.35 100.35 100.34 100.34 100.34 100.34 100.34 100.34 100.34 100.34 100.34 100.34 100.34 100.34 100.34 100.34 100.34 100.34 100.34 100.34 100.34 100.34 100.34 100.34 100.34]
  Signal 2 : Outport  Tag=STV Outport
  wires:
  FromWs/1 -> Demux/1
  Demux/1 -> Signal 2/1

== system Rocket_Full_Simulation/Plant/Aerodynamics/Signal Builder ==
  Demux : Demux  Tag=STV Demux  Outputs=2
      settings: DisplayOption=none
  FromWs : FromWorkspace  Tag=STV FromWs  VariableName=tuvar
      SigBuilderData=|
      | common.afterFinalStr = 'Extrapolate'
      | common.sampleTime = 0
      | dataSet.timeRange = [0 10]
      | dataSet.name = 'Group 1'
      | sbobj.Groups.Name = 'Group 1'
      | sbobj.Groups.Signals(1).Name = 'Logitudinal Moment of Inertia'
      | sbobj.Groups.Signals(1).XData = [0 0.01 0.02 0.03 0.04 0.05 0.06 0.07 0.08 0.09 0.1 0.11 0.12 0.13 0.14 0.15 0.16 0.17 0.18 0.19 0.2 0.21 0.22 0.23 0.24 0.25 0.26 0.27 0.28 0.29 0.3 0.31 0.32 0.33 0.34 0.35 0.36 0.37 0.38 0.39 0.4 0.41 0.42 0.43 0.44 0.455 0.4775 0.51125 0.56125 0.61125 0.66125 0.71125 0.76125 0.81125 0.86125 0.91125 0.95226 0.98929 1.029 1.0781 1.1281 1.1781 1.2281 1.2662 1.3014 1.342 1.392 1.442 1.492 1.5386 1.5886 1.6386 1.6886 1.7386 1.7886 1.8386 1.8886 1.9386 1.9886 2.0386 2.0886 2.1386 2.1886 2.2386 2.2886 2.3386 2.3886 2.4386 2.4886 2.5386 2.5886 2.6386 2.6886 2.7386 2.7886 2.8386 2.8886 10]
      | sbobj.Groups.Signals(1).YData = [0.81527 0.81527 0.81471 0.81406 0.81348 0.81295 0.81241 0.81188 0.81134 0.8108 0.81027 0.80973 0.80919 0.80866 0.80812 0.80758 0.80704 0.8065 0.80596 0.80542 0.80488 0.80434 0.8038 0.80326 0.80272 0.80217 0.80163 0.80109 0.80054 0.8 0.79946 0.79891 0.79836 0.79782 0.79727 0.79673 0.79618 0.79563 0.79508 0.79452 0.79397 0.79342 0.79286 0.79231 0.79175 0.79106 0.79001 0.78844 0.7861 0.7833 0.78048 0.77765 0.77488 0.77216 0.76943 0.76674 0.76432 0.76223 0.76018 0.7578 0.75514 0.75254 0.75002 0.74792 0.74634 0.74477 0.7431 0.74164 0.74043 0.73955 0.7389 0.73835 0.73798 0.73771 0.73753 0.73742 0.73734 0.7373 0.7373 0.7373 0.7373 0.7373 0.7373 0.7373 0.7373 0.7373 0.7373 0.7373 0.7373 0.7373 0.7373 0.7373 0.7373 0.7373 0.7373 0.7373 0.7373 0.7373]
      | sbobj.Groups.Signals(2).Name = 'Rotational Moment of Inertia'
      | sbobj.Groups.Signals(2).XData = [0 0.01 0.02 0.03 0.04 0.05 0.06 0.07 0.08 0.09 0.1 0.11 0.12 0.13 0.14 0.15 0.16 0.17 0.18 0.19 0.2 0.21 0.22 0.23 0.24 0.25 0.26 0.27 0.28 0.29 0.3 0.31 0.32 0.33 0.34 0.35 0.36 0.37 0.38 0.39 0.4 0.41 0.42 0.43 0.44 0.455 0.4775 0.51125 0.56125 0.61125 0.66125 0.71125 0.76125 0.81125 0.86125 0.91125 0.95226 0.98929 1.029 1.0781 1.1281 1.1781 1.2281 1.2662 1.3014 1.342 1.392 1.442 1.492 1.5386 1.5886 1.6386 1.6886 1.7386 1.7886 1.8386 1.8886 1.9386 1.9886 2.0386 2.0886 2.1386 2.1886 2.2386 2.2886 2.3386 2.3886 2.4386 2.4886 2.5386 2.5886 2.6386 2.6886 2.7386 2.7886 2.8386 2.8886 10]
      | sbobj.Groups.Signals(2).YData = [0.010422 0.010422 0.010421 0.010421 0.010421 0.010421 0.010421 0.010421 0.010421 0.01042 0.01042 0.01042 0.01042 0.01042 0.01042 0.01042 0.010419 0.010419 0.010419 0.010419 0.010419 0.010419 0.010419 0.010418 0.010418 0.010418 0.010418 0.010418 0.010418 0.010418 0.010417 0.010417 0.010417 0.010417 0.010417 0.010417 0.010417 0.010416 0.010416 0.010416 0.010416 0.010416 0.010416 0.010416 0.010415 0.010415 0.010415 0.010415 0.010414 0.010413 0.010413 0.010412 0.010411 0.01041 0.01041 0.010409 0.010408 0.010408 0.010407 0.010407 0.010406 0.010406 0.010405 0.010404 0.010404 0.010404 0.010403 0.010403 0.010403 0.010402 0.010402 0.010402 0.010402 0.010402 0.010402 0.010402 0.010402 0.010402 0.010402 0.010402 0.010402 0.010402 0.010402 0.010402 0.010402 0.010402 0.010402 0.010402 0.010402 0.010402 0.010402 0.010402 0.010402 0.010402 0.010402 0.010402 0.010402 0.010402]
  Logitudinal Moment of Inertia : Outport  Tag=STV Outport
  Rotational Moment of Inertia : Outport  Tag=STV Outport  Port=2
  wires:
  Demux/1 -> Logitudinal Moment of Inertia/1
  FromWs/1 -> Demux/1
  Demux/2 -> Rotational Moment of Inertia/1

== system Rocket_Full_Simulation/Plant/Overall Rocket/Impulse ==
  Demux : Demux  Tag=STV Demux  Outputs=1
      settings: DisplayOption=none
  FromWs : FromWorkspace  Tag=STV FromWs  VariableName=tuvar
      SigBuilderData=|
      | common.afterFinalStr = 'Extrapolate'
      | common.sampleTime = 0
      | dataSet.timeRange = [0 10]
      | dataSet.name = 'Group 1'
      | sbobj.Groups.Name = 'Group 1'
      | sbobj.Groups.Signals.Name = 'Signal 2'
      | sbobj.Groups.Signals.XData = [0 0.008 0.028 0.36 0.711 0.861 1.121 1.146 1.242 1.349 1.404 1.489 1.602 1.712 1.787 1.892 10]
      | sbobj.Groups.Signals.YData = [0 377.299 241.932 256.333 246.252 233.292 230.411 214.571 211.69 141.127 125.286 72.004 41.762 11.521 12.961 0 0]
  Signal 2 : Outport  Tag=STV Outport
  wires:
  FromWs/1 -> Demux/1
  Demux/1 -> Signal 2/1

== system Rocket_Full_Simulation/Plant/Overall Rocket/Mass ==
  Demux : Demux  Tag=STV Demux  Outputs=1
      settings: DisplayOption=none
  FromWs : FromWorkspace  Tag=STV FromWs  VariableName=tuvar
      SigBuilderData=|
      | common.afterFinalStr = 'Extrapolate'
      | common.sampleTime = 0
      | dataSet.timeRange = [0 10]
      | dataSet.name = 'Group 1'
      | sbobj.Groups.Name = 'Group 1'
      | sbobj.Groups.Signals.Name = 'Signal 2'
      | sbobj.Groups.Signals.XData = [0 0.01 0.02 0.03 0.04 0.05 0.06 0.07 0.08 0.09 0.1 0.11 0.12 0.13 0.14 0.15 0.16 0.17 0.18 0.19 0.2 0.21 0.22 0.23 0.24 0.25 0.26 0.27 0.28 0.29 0.3 0.31 0.32 0.33 0.34 0.35 0.36 0.37 0.38 0.39 0.4 0.41 0.42 0.43 0.44 0.455 0.4775 0.51125 0.56125 0.61125 0.66125 0.71125 0.76125 0.81125 0.86125 0.91106 0.9513 0.99131 1.0337 1.0837 1.1337 1.1837 1.2337 1.2765 1.3167 1.3643 1.4143 1.4643 1.5143 1.556 1.606 1.656 1.706 1.756 1.8028 1.8528 1.9028 1.9528 2.0028 2.0528 2.1028 2.1528 2.2028 2.2528 2.3028 2.3528 2.4028 2.4528 2.5028 2.5528 2.6028 2.6528 2.7028 2.7528 2.8028 2.8528 10]
      | sbobj.Groups.Signals.YData = [3464.9 3464.9 3463.5 3461.9 3460.4 3459 3457.7 3456.3 3455 3453.6 3452.3 3450.9 3449.6 3448.2 3446.9 3445.5 3444.2 3442.8 3441.5 3440.1 3438.8 3437.4 3436 3434.7 3433.3 3432 3430.6 3429.3 3427.9 3426.6 3425.2 3423.9 3422.5 3421.2 3419.8 3418.5 3417.1 3415.8 3414.4 3413 3411.7 3410.3 3408.9 3407.6 3406.2 3404.5 3402 3398.1 3392.4 3385.6 3378.8 3372 3365.3 3358.8 3352.3 3345.9 3340.2 3335.2 3330 3324.2 3317.9 3311.9 3306.1 3301.1 3297 3293 3289.2 3286.1 3283.7 3282 3280.6 3279.5 3278.8 3278.3 3278 3277.7 3277.6 3277.5 3277.5 3277.5 3277.5 3277.5 3277.5 3277.5 3277.5 3277.5 3277.5 3277.5 3277.5 3277.5 3277.5 3277.5 3277.5 3277.5 3277.5 3277.5 3277.5]
  Signal 2 : Outport  Tag=STV Outport
  wires:
  FromWs/1 -> Demux/1
  Demux/1 -> Signal 2/1

== matlab function Rocket_Full_Simulation/Plant/Aerodynamics/Airframe/Fins Stage 1 ==
  data: C_P_f1 output size=1; C_N_f1 output size=2; C_A_f1 output size=2; AoA input; d_bt input; Re input
function [C_P_f1, C_N_f1, C_A_f1]  = fcn(AoA, d_bt,Re) %only for trapezoidal fins
[C_N_f1, C_P_f1, C_A_f1] = Fins_Stage_1_Coefficients(d_bt, AoA, Re);

== matlab function Rocket_Full_Simulation/Plant/Overall Rocket/If_on_rail_don't_change ==
  data: Angles input; XYZ_Coords input; Angles_real output; change output
function [Angles_real, change] = fcn(Angles, XYZ_Coords)
[Angles_real, change] = If_on_rail_dont_change(XYZ_Coords, Angles);

== matlab function Rocket_Full_Simulation/Plant/Overall Rocket/Combine Forces and Convert to Cartesian ==
  data: XYZ_Inertial_Force input; Cart_Accel output; DCM input; Inertial_Accel_New output; Impulse input; Mass input
function [Cart_Accel,Inertial_Accel_New] = fcn(XYZ_Inertial_Force, DCM, Impulse, Mass)
[Cart_Accel, Inertial_Accel_New] = Combine_Forces_and_Convert_to_Cartesian(XYZ_Inertial_Force, Impulse, Mass, DCM);

== matlab function Rocket_Full_Simulation/Plant/Aerodynamics/MATLAB Function1 ==
  data: AoA input; Solvable output
function Solvable = fcn(AoA)
if abs(AoA) > deg2rad(15)
    Solvable = 0;
else
    Solvable = 1;
end

== matlab function Rocket_Full_Simulation/Plant/Aerodynamics/Air Properties/MATLAB Function ==
  settings: updateMethod=CONTINUOUS  sampleTime=0.1
  data: t input; p input; rho output; h input; nu output
function [rho,nu] = AirDensityViscosity(t, p, h)



% AirProperties calculates a variety of air thermodynamic properties from 
% measured values of temperature, pressure and humidity. 
% 
% Variables able to calcuated: 
%   rho         [kg m^-3]       Density
%   mu          [N s m^-2]      Dynamic viscosity
%   k           [W m^-1 K^-1]   Thermal conductivity
%   c_p         [J kg^-1 K^-1]  Specific heat capacity (constant pressure)
%   c_v         [J kg^-1 K^-1]  Specific heat capacity (constant volume)
%   gamma       [1]             Ratio of specific heats
%   c           [m s^-1]        Speed of sound: c = (gamma*R*T/M)^0.5
%   nu          [m^2 s^-1]      Kinematic viscosity: nu = mu/rho
%   alpha       [m^2 s^-1]      Thermal diffusivity: alpha = k/(rho*c_p)
%   Pr          [1]             Prandtl number: Pr = mu*c_p/k
%   M           [kg mol^-1]     Molar mass of humid air
%   R           [J kg^-1 K^-1]  Specific gas constant
%   h           [%]             Relative humidity (if dewpoint inputted)
% 
% Syntax
%   rho = AirProperties
%   [...] = AirProperties(t, p)
%   [...] = AirProperties(t, p, h)
%   [...] = AirProperties(t, p, t_dp, 'DewPoint')
%   [...] = AirProperties(t, p, [], ...)
%   [...] = AirProperties(..., 'xCO2',0.0005)
%   [..., rho]     = AirProperties(..., 'rho')
%   [..., mu]      = AirProperties(..., 'mu')
%   [..., k]       = AirProperties(..., 'k')
%   [..., c_p]     = AirProperties(..., 'c_p')
%   [..., c_v]     = AirProperties(..., 'c_v')
%   [..., gamma]   = AirProperties(..., 'gamma')
%   [..., c]       = AirProperties(..., 'c')
%   [..., nu]      = AirProperties(..., 'nu')
%   [..., alpha]   = AirProperties(..., 'alpha')
%   [..., Pr]      = AirProperties(..., 'Pr')
%   [..., M]       = AirProperties(..., 'M')
%   [..., R]       = AirProperties(..., 'R')
%   [..., h]       = AirProperties(..., 'h')
%   [rho, mu, k, c_p, c_v, gamma, c, nu, alpha, Pr, M, R, h] = AirProperties(t, p, h)
% 
% Inputs
%   <None>      If no inputs are given then it returns the ISA standard air
%               density at 1013.25 hPa and 15°C: 1.225 [kg m^-3].
%               (Recommended value range - see references.)
%   t           ( 15 <= t <= 27  ) [°C]     (m x 1 numeric) Air temperature.
%   p           (600 <= p <= 1100) [hPa]    (m x 1 numeric) Air pressure.
%                   If the pressure is unknown, input [] as p and calculations 
%                   will proceed assuming the standard atmosphere (1013.25 hPa)
%   h           (  0 <= h <= 100 ) [%]      (m x 1 numeric) Relative humidity.
%                   If the humidity is unknown, input [] as h and calculations 
%                   will proceed assuming dry air. 
% 
% Inputs (Optional) 
%   'DewPoint'  Option to calculate the air properties with the dew point rather
%               than the relative humidity. This uses the third input as the 
%               value for dewpoint: t_dp [°C] (t_dp <= t) (m x 1 numeric)
%   'xCO2'      [mol mol^-1] (1 x 1 numeric) Mole fraction of CO2 in the air.
%               Used to improve the estimate of the molar mass of dry air.
%               Default 0.0004.
%   <Output>    (char) The variable to output. 
%               The order of the outputs will follow the input order. 
%               If none of these are provided then the outputs will follow the 
%               default order up to the number of outputs requested (nargout).
%               One or more of the above listed variables. 
% 
% Example Usage
%   rho = AirProperties
%   rho = AirProperties(18)
%   rho = AirProperties(18, 1010)
%   rho = AirProperties(18, 1010, 45)
%   [rho, mu, k] = AirProperties(22, 1010, 18, 'Dewpoint')
%   [rho, mu, k] = AirProperties(18, 1010, 45, 'xCO2', 0.0005)
%   [rho, mu, nu, c] = AirProperties(18, 1010, 45, 'rho', 'mu', 'nu', 'c')
%   [c, nu, mu, rho] = AirProperties(18, 1010, 45, 'c', 'nu', 'mu', 'rho')
%   [c, nu, mu, rho] = AirProperties(18, 1010, [], 'c', 'nu', 'mu', 'rho')
%   [c, nu, mu, rho] = AirProperties(18,   [], [], 'c', 'nu', 'mu', 'rho')
%   
%   t = (15:25)';   p = 1010;           h = 40; 
%   t = 25;         p = (950:10:1040)'; h = 40; 
%   t = 25;         p = 1010;           h = (0:10:100)'; 
%   t = linspace(15,25,10)'; p=linspace(950,1040,10)'; h=linspace(0,100,10)';
%   [rho, mu, k, c, c_p] = AirProperties(t, p, h, 'rho', 'mu', 'k', 'c', 'c_p')
% 
%   t = 0:100; p = 1013.25; h = 0:10:100;
%   n = length(h); Col = repmat((1-1/n:-1/n:0)', 1,3);
%   figure('Position',[50,50,500,400]); hold on; 
%   for ii = 1:n
%       rho(:,ii) = AirProperties(t, [], h(ii), 'rho');
%       plot(t, rho(:,ii), 'color',Col(ii,:));
%   end
%   annotation('textarrow',[0.8,0.75],[0.65,0.35],'String','Humidity')
%   xlabel('Temperature [°C]'); 
%   ylabel('\rho [kg m^{-3}]'); 
%   title('Density of air')
% 
% References:
%   Picard, A, Davis, RS, Glaser, M, Fujii, K, 2008, 'Revised formula for the
%   density of moist air (CIPM-2007)', Metrologia, vol. 45, no. 2, pp. 149-155.
%   DOI: http://dx.doi.org/10.1088/0026-1394/45/2/004
%
%   Tsilingiris, P, 2008, 'Thermophysical and transport properties of humid air
%   at temperature range between 0 and 100°C', Energy Conversion and
%   Management, vol. 49, no. 5, pp.1098-1110. 
%   DOI: https://doi.org/10.1016/j.enconman.2007.09.015
% 
% Shaun Fitzgerald
% Created 2017-09-25
% Modified 
%   2020-03-09  Included calculation of various extra air properties. 
%   2020-11-17  Added to GitHub
%% Inputs 
if nargin == 0
    % ISA standard density of air at 15 °C and 1013.25 hPa
    varout{1} = 1.225;           % [kg m^-3]
    return
end
% Temperature
assert(isnumeric(t) && isvector(t), ...
    'Expected input ''t'' to be a numeric vector or scalar.')
% Pressure
if nargin < 2 || isempty(p)
    p = 1013.25;                    % [hPa] (1 atm)
else
    assert(isnumeric(p) && isvector(p), ...
        'Expected input ''p'' to be a numeric vector or scalar.')
    assert(all(p >= 0), 'Cannot have a negative pressure.')
end
% Humidity
if nargin < 3 || isempty(h)
    UseHumidity = false;
else
    UseHumidity = true;
    assert(isnumeric(h) && isvector(h), ...
        'Expected input ''h'' to be a numeric vector or scalar.')
    assert(all(h >= 0) && all(h <= 100), ...
        'The humidity must be in the range: 0 <= h <= 100.')
end
% Default values
xCO2        = 0.0004;
DewPoint    = false;


%% Basic calculations 
% Constants
R  = 8.314472;                                  % [J mol^-1 K^-1]   Gas Constant
Ma = (28.96546 + 12.011*(xCO2 - 0.0004))*1e-3;  % [kg mol^-1]       Dry air
Mv = 18.01528e-3;                               % [kg mol^-1]       Water Vapour

%% Humidity 
if UseHumidity
    % Saturation vapour pressure
    A =  1.2378847e-5;                          % [K^-2]
    B = -1.9121316e-2;                          % [K^-1]
    C = 33.93711047;                            % [1]
    D = -6.3431645e3;                           % [K]
    p_sv = exp(A*t.^2 + B*t + C + D./t);        % [Pa]
    
    % Enhancement factor
    alpha = 1.00062;                            % [1]
    beta  = 3.14e-8;                            % [Pa^-1]
    gamma = 5.6e-7;                             % [K^-2]
    f = alpha + beta*p + gamma*t.^2;            % [1]
    
    % Mole fraction of water vapour
    if DewPoint    % With dew point temperature
        t_dp = h;
        if any(t_dp > t)
            error('The dew point cannot be greater than the temperature.')
        end
        
        f_dp = alpha + beta*p + gamma*t_dp.^2;  % [1]
        x_v = f_dp.*p_sv./p;                    % [1]
        
        % Calculating relative humidity
        T_dp = t_dp + 273.15;                   % [K]
        p_sv_dp = exp(A*T_dp.^2 + B*T_dp + C + D./T_dp);  % [Pa]
        H = p_sv_dp.*f_dp./(p_sv.*f);           % [1]
        
    else           % With relative humidity
        H = h./100;                             % [1]
        x_v = H.*f.*p_sv./p;                    % [1]
        
    end
    
    % Molar mass of humid air
    M = Ma*(1 - x_v) + Mv*x_v;                  % [kg mol^-1]
    
    % Compressibility Factor
    a0 =  1.58123e-6;                           % [K Pa^-1]
    a1 = -2.93310e-8;                           % [Pa^-1]
    a2 =  1.10430e-10;                          % [K^-1 Pa^-1]
    b0 =  5.70700e-6;                           % [K Pa^-1]
    b1 = -2.05100e-8;                           % [Pa^-1]
    c0 =  1.98980e-4;                           % [K Pa^-1]
    c1 = -2.37600e-6;                           % [Pa^-1]
    d  =  1.83000e-11;                          % [K^2 Pa^-2]
    e  = -0.76500e-8;                           % [K^2 Pa^-2]
    
    Z = 1 - p./t.*(a0 + a1*t + a2*t.^2 + (b0 + b1*t).*x_v + ...
        (c0 + c1*t).*x_v.^2) + p.^2.*t.^-2.*(d + e*x_v.^2);    % [1]
else
    
        OutputNum.h = NaN;
    
    
    % Assuming the molar mass of dry air
    M = Ma;                                     % [kg mol^-1]
    Z = 1;                                      % [1]
end
%% Density & molecular values
rho = p.*M./(R*Z.*t);                           % [kg m^-3]


%% Viscosity 

% Dry air - for 250 <= T <= 600 K
MA0 = -9.8601e-1;
MA1 =  9.080125e-2;
MA2 = -1.17635575e-4;
MA3 =  1.2349703e-7;
MA4 = -5.7971299e-11;
mu_a = (MA0 + MA1*t + MA2*t.^2 + MA3*t.^3 + MA4*t.^4)*1e-6; % [N s m^-2]

if UseHumidity
    % Water vapour - for 0 <= t <= 120 °C
    MV0 = 80.58131868;
    MV1 =  0.4000549451;
    mu_v = (MV0 + MV1*t)*1e-7;              % [N s m^-2]

    % Interaction parameters
    Phi_av = 2^0.5/4*(1+Ma/Mv)^-0.5.*(1+(mu_a./mu_v).^0.5*(Mv/Ma)^0.25).^2;
    Phi_va = 2^0.5/4*(1+Mv/Ma)^-0.5.*(1+(mu_v./mu_a).^0.5*(Ma/Mv)^0.25).^2;

    % Mixture viscosity
    mu = ((1 - x_v).*mu_a)./((1 - x_v) + x_v.*Phi_av) + ...
        (x_v.*mu_v)./(x_v + (1 - x_v).*Phi_va); % [N s m^-2]
else
    mu = mu_a;
end

          % [N s m^-2]


% Kinematic viscosity

nu = mu./rho;                           % [m^2 s^-1]

== matlab function Rocket_Full_Simulation/Plant/Aerodynamics/Airframe/Body  and Nosecone Coefficients ==
  data: NC_Base_A output; C_P_B output size=1; C_P_NC output size=1; C_N_B output size=2; C_N_NC output size=2; C_A_BN output size=2; L_N input; L_B input; L_C input; D_B input; D_D input; Re input; AoA input; Nu input; K input
function [NC_Base_A,C_P_B,C_P_NC,C_N_B,C_N_NC,C_A_BN] = Coefficients(L_N, L_B, L_C, D_B, D_D, Re, AoA, Nu, K)
[NC_Base_A, C_N_B, C_N_NC, C_A_BN, C_P_NC, C_P_B] = Body_and_Nosecone_Coefficients(Re, L_N, L_B, D_B, D_D, L_C, AoA, Nu, K);

== matlab function Rocket_Full_Simulation/Simulation/MATLAB Function ==
  data: Rotation output; Angles input
function Rotation  = fcn(Angles)

Rotation = [sin(Angles(2))*cos(Angles(1)); 
              cos(Angles(2))*cos(Angles(1));
              sin(Angles(1));
              Angles(3)];

== matlab function Rocket_Full_Simulation/Plant/Aerodynamics/Airframe/Flaps ==
  data: C_P_flaps output size=1; C_N_flaps output size=2; AoA input; AoA_flaps input; d_bt input; C_A_flaps output size=2; Re input; C_N_roll output size=1
function [C_P_flaps,C_N_flaps,C_A_flaps,C_N_roll] = fcn(AoA,AoA_flaps,d_bt,Re) %only for trapezoidal fins
[C_N_flaps, C_N_roll, C_P_flaps, C_A_flaps] = Active_Fins_Coefficients(d_bt, AoA, AoA_flaps, Re);

== matlab function Rocket_Full_Simulation/Plant/Aerodynamics/MATLAB Function ==
  data: AoA input; Solvable output
function Solvable = fcn(AoA)
if abs(AoA) > deg2rad(15)
    Solvable = 0;
else
    Solvable = 1;
end

== matlab function Rocket_Full_Simulation/Plant/Overall Rocket/Calculate AoA and Vel_Magn ==
  data: AoA output; Cart_Vel input; Vel_Magn output; DCM input; Angles input; Inertial_Vel output
function [AoA,Vel_Magn,Inertial_Vel] = fcn(Cart_Vel, DCM, Angles)
[Vel_Magn, Inertial_Vel, AoA] = Calculate_AoA_and_Vel_Magn(Cart_Vel, DCM, Angles);

== matlab function Rocket_Full_Simulation/Plant/Aerodynamics/Airframe/Fins Stage 2 ==
  data: C_P_f2 output size=1; C_N_f2 output size=2; AoA input; d_bt input; C_A_f2 output size=2; Re input
function [C_P_f2,C_N_f2,C_A_f2] = fcn(AoA, d_bt,Re) %only for trapezoidal fins
[C_N_f2, C_P_f2, C_A_f2] = Fins_Stage_2_Coefficients(d_bt, AoA, Re);
